simulink model "eq_inertia_torque"  (R2023b)
settings: Solver=VariableStepAuto  StartTime=0.0  StopTime=10.0  RelTol=1e-3
values from neighbouring files (symbols this model uses):
  g = 9.81    [ElevatorAndMotorTemplate.m]
  i = ?    [ElevatorAndMotorTemplate.m]
  r = ?    [ElevatorAndMotorTemplate.m]
settings Model: Creator=alalar1  LastModifiedBy=alalar1

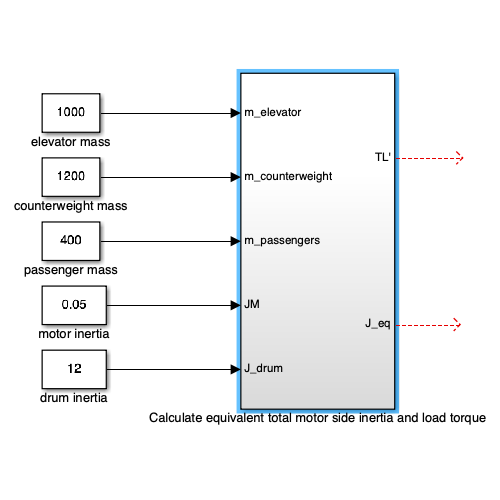
[thumbnail: Simulink's stored preview of the top-level diagram]
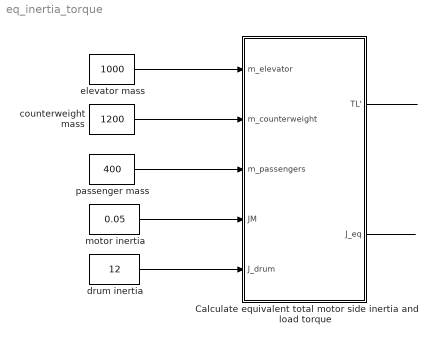
== system eq_inertia_torque ==
  Calculate equivalent total motor side inertia and load torque : Subsystem
  counterweight mass : Constant  Value=1200
  drum inertia : Constant  Value=12
  elevator mass : Constant  Value=1000
  motor inertia : Constant  Value=0.05
  passenger mass : Constant  Value=400
  wires:
  drum inertia/1 -> Calculate equivalent total motor side inertia and load torque/5(J_drum)
  counterweight mass/1 -> Calculate equivalent total motor side inertia and load torque/2(m_counterweight)
  motor inertia/1 -> Calculate equivalent total motor side inertia and load torque/4(JM)
  passenger mass/1 -> Calculate equivalent total motor side inertia and load torque/3(m_passengers)
  elevator mass/1 -> Calculate equivalent total motor side inertia and load torque/1(m_elevator)
  Calculate equivalent total motor side inertia and load torque/1(TL') -> ?
  Calculate equivalent total motor side inertia and load torque/2(J_eq) -> ?

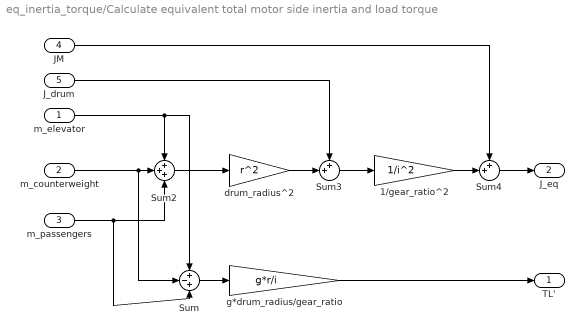
== system eq_inertia_torque/Calculate equivalent total motor side inertia and load torque ==
  m_elevator : Inport
  m_counterweight : Inport  Port=2
  m_passengers : Inport  Port=3
  JM : Inport  Port=4
  J_drum : Inport  Port=5
  1/gear_ratio^2 : Gain  Gain=1/i^2
  Sum : Sum  Inputs=+-+
  Sum2 : Sum  Inputs=+++
  Sum3 : Sum  Inputs=++|
  Sum4 : Sum  Inputs=++|
  drum_radius^2 : Gain  Gain=r^2
  g*drum_radius/gear_ratio : Gain  Gain=g*r/i
  TL' : Outport
  J_eq : Outport  Port=2
  wires:
  m_elevator/1 -> Sum/1, Sum2/1
  drum_radius^2/1 -> Sum3/2
  m_passengers/1 -> Sum2/3, Sum/3
  Sum2/1 -> drum_radius^2/1
  JM/1 -> Sum4/1
  J_drum/1 -> Sum3/1
  Sum3/1 -> 1/gear_ratio^2/1
  m_counterweight/1 -> Sum/2, Sum2/2
  1/gear_ratio^2/1 -> Sum4/2
  Sum4/1 -> J_eq/1
  Sum/1 -> g*drum_radius/gear_ratio/1
  g*drum_radius/gear_ratio/1 -> TL'/1
